simulink model "Boeing787_NewMission_ElectricalThermalHydraulicECS"  (R2016a)
settings: Solver=ode23tb  SolverMode=SingleTasking  StartTime=0.0  StopTime=346  RelTol=1e-3
InitFcn:
  | load('SampleOutput.mat')
  | 
  | load('SampleFuelBurn.mat')
undefined symbols (not defined in the file): ailerons, AirProp, B_737, CurrentMission, elevator, FuelBurn, HydProp, landing_gear, rudder, seed, thrust_rev
libraries: PowerFlowLib x68, simulink x20, powerlib_meascontrol x1
(part 18 of 24)

== system Boeing787_NewMission_ElectricalThermalHydraulicECS/Hydraulic/Center Hydraulic System/Bootstrap Reservoir1 ==
  Piston Pressure : Inport
  Bypass Return : Inport  Port=2
  mdot_out : Inport  Port=3
  Return : Inport  Port=4
  Add : Sum  Inputs=+-
  Bleed Valve on/off : Switch  Criteria=u2 ~= 0  ZeroCross=off
  Bleed Valve on/off1 : Switch  Criteria=u2 > Threshold  ZeroCross=off
  Bus Creator : BusCreator  Inputs=2
  Bus Creator1 : BusCreator  Inputs=3
  Bus Creator2 : BusCreator  Inputs=3
  Bus Selector2 : BusSelector  OutputSignals=pres_kPa
  Bus Selector3 : BusSelector  OutputSignals=temp_K,mdot_kgps
  Bus Selector4 : BusSelector  OutputSignals=pres_kPa,mdot_kgps,temp_K
  Divide : Product  Inputs=****/
  Divide1 : Product  Inputs=**/
  Divide2 : Product  Inputs=/*
  Divide3 : Product  Inputs=**
  Divide4 : Product  Inputs=**
  Gain : Gain  Gain=1/1000
  Gain1 : Gain  Gain=pres_loss/100
  Gain{2..7} (6 alike) : Gain
  R_air : Constant  Value=286.9
  Relational Operator : RelationalOperator  OutDataTypeStr=boolean
  Sum : Sum  Inputs=++-
  Sum of Elements : Sum  Inputs=+
  Sum1 : Sum  Inputs=|+-
  Sum2 : Sum  Inputs=-+|
  Sum3 : Sum  Inputs=-+|
  Sum4 : Sum  Inputs=|++
  Temp : Integrator  InitialCondition=T_init  LimitOutput=on  LowerSaturationLimit=eps
  Terminator : Terminator
  Terminator1 : Terminator
  Z(T,P) : Lookup_n-D  BreakpointsForDimension1=AirProp.T2  BreakpointsForDimension2=AirProp.P2  Table=AirProp.Z  RndMeth=Simplest  InputSameDT=on
  air pres : Integrator  InitialCondition=P_init*1000
  mass : Integrator  InitialCondition=mass_init  LimitOutput=on  LowerSaturationLimit=eps
  mass flow off{,1,7..9} (5 alike) : Constant  Value=0
  mass flow off10 : Constant  Value=T_init
  mass flow off2 : Constant  Value=High_Pres_Area
  mass flow off3 : Constant  Value=Low_Pres_Area
  mass flow off4 : Constant  Value=10
  mass flow off5 : Constant  Value=275.79
  mass flow off6 : Constant  Value=-10
  resevor volume : Constant  Value=res_vol
  rho(T) : Lookup_n-D  NumberOfTableDimensions=1  BreakpointsForDimension1=HydProp.T  Table=HydProp.rho_T  RndMeth=Simplest  InputSameDT=on
  Fluid Conditions : Outport
  wires:
  Piston Pressure/1 -> Sum4/1, Divide3/1
  mass flow off1/1 -> Bleed Valve on/off/3
  Divide2/1 -> Sum1/2
  rho(T)/1 -> Divide2/1
  Sum of Elements/1 -> Sum/2
  Return/1 -> Sum of Elements/1
  mass flow off10/1 -> Gain5/1
  Temp/1 -> rho(T)/1, Sum3/1  "temp_K"
  Sum3/1 -> Divide1/1
  Divide1/1 -> Temp/1
  mass/1 -> Divide1/3, Divide2/2
  Bus Creator1/1 -> Fluid Conditions/1
  [valve_cmd] -> Bleed Valve on/off/2
  Relational Operator/1 -> [valve_cmd]
  mass flow off/1 -> Bleed Valve on/off/1
  Bus Selector2/1 -> Relational Operator/1  "<pres_kPa>"
  Bus Selector4/1 -> Relational Operator/2  "<pres_kPa>"
  Bleed Valve on/off/1 -> Terminator1/1, Gain1/1, Sum2/2
  Bus Selector4/2 -> Terminator/1  "<mdot_kgps>"
  Sum2/1 -> Divide/2  "dm/dt"
  Bus Creator/1 -> Bus Selector2/1
  Gain1/1 -> Sum2/1, Bus Creator/1  "mdot_kgps"
  Gain/1 -> Bus Creator/2, Z(T,P)/2  "pres_kPa"
  Sum1/1 -> Divide/5
  resevor volume/1 -> Sum1/1
  air pres/1 -> Gain/1
  Divide/1 -> air pres/1
  Z(T,P)/1 -> Divide/4
  R_air/1 -> Divide/1
  Bus Selector4/3 -> Divide/3, Z(T,P)/1  "<temp_K>"
  Sum/1 -> mass/1  "dm/dt"
  mdot_out/1 -> Gain6/1, Sum/3  "mdot_kgps"
  Bus Selector3/2 -> Sum/1, Divide1/2  "<mdot_kgps>"
  Bypass Return/1 -> Bus Selector3/1
  mass flow off2/1 -> Divide3/2
  mass flow off3/1 -> Divide4/2
  mass flow off5/1 -> Divide4/1
  Divide4/1 -> Add/2
  Divide3/1 -> Add/1
  Add/1 -> Bleed Valve on/off1/2
  mass flow off6/1 -> Bleed Valve on/off1/3
  Bleed Valve on/off1/1 -> Sum4/2
  mass flow off4/1 -> Bleed Valve on/off1/1  "pres_kPa"
  Bus Creator2/1 -> Bus Selector4/1
  mass flow off9/1 -> Gain4/1
  mass flow off8/1 -> Gain3/1
  mass flow off7/1 -> Gain2/1
  Gain2/1 -> Bus Creator2/1  "pres_kPa"
  Gain4/1 -> Bus Creator2/3  "temp_K"
  Gain3/1 -> Bus Creator2/2  "mdot_kgps"
  Gain6/1 -> Bus Creator1/3  "mdot_kgps"
  Gain5/1 -> Bus Creator1/2  "temp_K"
  Sum4/1 -> Gain7/1  "pres_kPa"
  Gain7/1 -> Bus Creator1/1  "pres_kPa"

== system Boeing787_NewMission_ElectricalThermalHydraulicECS/Hydraulic/Center Hydraulic System/Bootstrap Reservoir2 ==
  Piston Pressure : Inport
  Bypass Return : Inport  Port=2
  mdot_out : Inport  Port=3
  Return : Inport  Port=4
  Add : Sum  Inputs=+-
  Bleed Valve on/off : Switch  Criteria=u2 ~= 0  ZeroCross=off
  Bleed Valve on/off1 : Switch  Criteria=u2 > Threshold  ZeroCross=off
  Bus Creator : BusCreator  Inputs=2
  Bus Creator1 : BusCreator  Inputs=3
  Bus Creator2 : BusCreator  Inputs=3
  Bus Selector2 : BusSelector  OutputSignals=pres_kPa
  Bus Selector3 : BusSelector  OutputSignals=temp_K,mdot_kgps
  Bus Selector4 : BusSelector  OutputSignals=pres_kPa,mdot_kgps,temp_K
  Divide : Product  Inputs=****/
  Divide1 : Product  Inputs=**/
  Divide2 : Product  Inputs=/*
  Divide3 : Product  Inputs=**
  Divide4 : Product  Inputs=**
  Gain : Gain  Gain=1/1000
  Gain1 : Gain  Gain=pres_loss/100
  Gain{2..7} (6 alike) : Gain
  R_air : Constant  Value=286.9
  Relational Operator : RelationalOperator  OutDataTypeStr=boolean
  Sum : Sum  Inputs=++-
  Sum of Elements : Sum  Inputs=+
  Sum1 : Sum  Inputs=|+-
  Sum2 : Sum  Inputs=-+|
  Sum3 : Sum  Inputs=-+|
  Sum4 : Sum  Inputs=|++
  Temp : Integrator  InitialCondition=T_init  LimitOutput=on  LowerSaturationLimit=eps
  Terminator : Terminator
  Terminator1 : Terminator
  Z(T,P) : Lookup_n-D  BreakpointsForDimension1=AirProp.T2  BreakpointsForDimension2=AirProp.P2  Table=AirProp.Z  RndMeth=Simplest  InputSameDT=on
  air pres : Integrator  InitialCondition=P_init*1000
  mass : Integrator  InitialCondition=mass_init  LimitOutput=on  LowerSaturationLimit=eps
  mass flow off{,1,7..9} (5 alike) : Constant  Value=0
  mass flow off2 : Constant  Value=High_Pres_Area
  mass flow off3 : Constant  Value=Low_Pres_Area
  mass flow off4 : Constant  Value=10
  mass flow off5 : Constant  Value=275.79
  mass flow off6 : Constant  Value=-10
  resevor volume : Constant  Value=res_vol
  rho(T) : Lookup_n-D  NumberOfTableDimensions=1  BreakpointsForDimension1=HydProp.T  Table=HydProp.rho_T  RndMeth=Simplest  InputSameDT=on
  Fluid Conditions : Outport
  wires:
  Piston Pressure/1 -> Sum4/1, Divide3/1
  mass flow off1/1 -> Bleed Valve on/off/3
  Divide2/1 -> Sum1/2
  rho(T)/1 -> Divide2/1
  Sum of Elements/1 -> Sum/2
  Return/1 -> Sum of Elements/1
  Bus Selector3/1 -> Gain5/1  "<temp_K>"
  Temp/1 -> rho(T)/1, Sum3/1  "temp_K"
  Sum3/1 -> Divide1/1
  Divide1/1 -> Temp/1
  mass/1 -> Divide1/3, Divide2/2
  Bus Creator1/1 -> Fluid Conditions/1
  [valve_cmd] -> Bleed Valve on/off/2
  Relational Operator/1 -> [valve_cmd]
  mass flow off/1 -> Bleed Valve on/off/1
  Bus Selector2/1 -> Relational Operator/1  "<pres_kPa>"
  Bus Selector4/1 -> Relational Operator/2  "<pres_kPa>"
  Bleed Valve on/off/1 -> Terminator1/1, Gain1/1, Sum2/2
  Bus Selector4/2 -> Terminator/1  "<mdot_kgps>"
  Sum2/1 -> Divide/2  "dm/dt"
  Bus Creator/1 -> Bus Selector2/1
  Gain1/1 -> Sum2/1, Bus Creator/1  "mdot_kgps"
  Gain/1 -> Bus Creator/2, Z(T,P)/2  "pres_kPa"
  Sum1/1 -> Divide/5
  resevor volume/1 -> Sum1/1
  air pres/1 -> Gain/1
  Divide/1 -> air pres/1
  Z(T,P)/1 -> Divide/4
  R_air/1 -> Divide/1
  Bus Selector4/3 -> Divide/3, Z(T,P)/1  "<temp_K>"
  Sum/1 -> mass/1  "dm/dt"
  mdot_out/1 -> Gain6/1, Sum/3  "mdot_kgps"
  Bus Selector3/2 -> Sum/1, Divide1/2  "<mdot_kgps>"
  Bypass Return/1 -> Bus Selector3/1
  mass flow off2/1 -> Divide3/2
  mass flow off3/1 -> Divide4/2
  mass flow off5/1 -> Divide4/1
  Divide4/1 -> Add/2
  Divide3/1 -> Add/1
  Add/1 -> Bleed Valve on/off1/2
  mass flow off6/1 -> Bleed Valve on/off1/3
  Bleed Valve on/off1/1 -> Sum4/2
  mass flow off4/1 -> Bleed Valve on/off1/1  "pres_kPa"
  Bus Creator2/1 -> Bus Selector4/1
  mass flow off9/1 -> Gain4/1
  mass flow off8/1 -> Gain3/1
  mass flow off7/1 -> Gain2/1
  Gain2/1 -> Bus Creator2/1  "pres_kPa"
  Gain4/1 -> Bus Creator2/3  "temp_K"
  Gain3/1 -> Bus Creator2/2  "mdot_kgps"
  Gain6/1 -> Bus Creator1/3  "mdot_kgps"
  Gain5/1 -> Bus Creator1/2  "temp_K"
  Sum4/1 -> Gain7/1  "pres_kPa"
  Gain7/1 -> Bus Creator1/1  "pres_kPa"

== system Boeing787_NewMission_ElectricalThermalHydraulicECS/Hydraulic/Center Hydraulic System/DC Speed Servo ==
  T_load (Nm) : Inport
  Speed_ref (RPM) : Inport  Port=2
  Voltage : Inport  Port=3
  DC Machine : Subsystem
  Fcn : Fcn  Expr=u(1)/(u(2)+0.1)
  Gain2 : Gain  Gain=60/(2*pi)
  Mux : Mux  Inputs=2
  PID Controller : simulink/Continuous/PID Controller  Controller=PID  TimeDomain=Continuous-time  SampleTime=-1  IntegratorMethod=Forward Euler  FilterMethod=Forward Euler  Form=Parallel  UseFilter=on  ControllerParametersSource=internal  P=1  I=0.1  D=0  N=100  InitialConditionSource=internal  InitialConditionForIntegrator=0  InitialConditionForFilter=0  ExternalReset=none  LimitOutput=off  UpperSaturationLimit=inf  LowerSaturationLimit=-inf  LinearizeAsGain=on  AntiWindupMode=none  Kb=1  TrackingMode=off  Kt=1  PParamMin=[]  PParamMax=[]  IParamMin=[]  IParamMax=[]  DParamMin=[]  DParamMax=[]  NParamMin=[]  NParamMax=[]  KbParamMin=[]  KbParamMax=[]  KtParamMin=[]  KtParamMax=[]  POutMin=[]  POutMax=[]  IOutMin=[]  IOutMax=[]  DOutMin=[]  DOutMax=[]  NOutMin=[]  NOutMax=[]  KbOutMin=[]  KbOutMax=[]  KtOutMin=[]  KtOutMax=[]  IntegratorOutMin=[]  IntegratorOutMax=[]  FilterOutMin=[]  FilterOutMax=[]  SumOutMin=[]  SumOutMax=[]  SumI1OutMin=[]  SumI1OutMax=[]  SumI2OutMin=[]  SumI2OutMax=[]  SumI3OutMin=[]  SumI3OutMax=[]  SumDOutMin=[]  SumDOutMax=[]  SaturationOutMin=[]  SaturationOutMax=[]  IntegratorContinuousStateAttributes=''  IntegratorStateMustResolveToSignalObject=off  IntegratorRTWStateStorageClass=Auto  FilterContinuousStateAttributes=''  FilterStateMustResolveToSignalObject=off  FilterRTWStateStorageClass=Auto  DifferentiatorICPrevScaledInput=0  DifferentiatorOutMin=[]  DifferentiatorOutMax=[]
  Sum : Sum  Inputs=-+|
  Terminator{,1..3} (4 alike) : Terminator
  w_m : Outport
  i_load : Outport  Port=2
  T_em : Outport  Port=3
  Ploss : Outport  Port=4
  wires:
  DC Machine/5(Plosses) -> Ploss/1
  Sum/1 -> PID Controller/1
  Gain2/1 -> Sum/1, w_m/1
  Speed_ref (RPM)/1 -> Sum/2
  T_load (Nm)/1 -> DC Machine/3(Tload)
  DC Machine/6(Te) -> T_em/1
  Mux/1 -> Fcn/1
  DC Machine/3(Pe) -> Mux/1
  Fcn/1 -> i_load/1
  DC Machine/7(Speed) -> Gain2/1
  Voltage/1 -> DC Machine/1(Vf), Mux/2
  PID Controller/1 -> DC Machine/2(Va)
  DC Machine/1(If) -> Terminator/1
  DC Machine/2(Ia) -> Terminator1/1
  DC Machine/4(Pm) -> Terminator2/1
  DC Machine/8(theta) -> Terminator3/1

== system Boeing787_NewMission_ElectricalThermalHydraulicECS/Hydraulic/Center Hydraulic System/DC Speed Servo1 ==
  T_load (Nm) : Inport
  Speed_ref (RPM) : Inport  Port=2
  Voltage : Inport  Port=3
  DC Machine : Subsystem
  Fcn : Fcn  Expr=u(1)/(u(2)+0.1)
  Gain2 : Gain  Gain=60/(2*pi)
  Mux : Mux  Inputs=2
  PID Controller : simulink/Continuous/PID Controller  Controller=PID  TimeDomain=Continuous-time  SampleTime=-1  IntegratorMethod=Forward Euler  FilterMethod=Forward Euler  Form=Parallel  UseFilter=on  ControllerParametersSource=internal  P=1  I=0.1  D=0  N=100  InitialConditionSource=internal  InitialConditionForIntegrator=0  InitialConditionForFilter=0  ExternalReset=none  LimitOutput=off  UpperSaturationLimit=inf  LowerSaturationLimit=-inf  LinearizeAsGain=on  AntiWindupMode=none  Kb=1  TrackingMode=off  Kt=1  PParamMin=[]  PParamMax=[]  IParamMin=[]  IParamMax=[]  DParamMin=[]  DParamMax=[]  NParamMin=[]  NParamMax=[]  KbParamMin=[]  KbParamMax=[]  KtParamMin=[]  KtParamMax=[]  POutMin=[]  POutMax=[]  IOutMin=[]  IOutMax=[]  DOutMin=[]  DOutMax=[]  NOutMin=[]  NOutMax=[]  KbOutMin=[]  KbOutMax=[]  KtOutMin=[]  KtOutMax=[]  IntegratorOutMin=[]  IntegratorOutMax=[]  FilterOutMin=[]  FilterOutMax=[]  SumOutMin=[]  SumOutMax=[]  SumI1OutMin=[]  SumI1OutMax=[]  SumI2OutMin=[]  SumI2OutMax=[]  SumI3OutMin=[]  SumI3OutMax=[]  SumDOutMin=[]  SumDOutMax=[]  SaturationOutMin=[]  SaturationOutMax=[]  IntegratorContinuousStateAttributes=''  IntegratorStateMustResolveToSignalObject=off  IntegratorRTWStateStorageClass=Auto  FilterContinuousStateAttributes=''  FilterStateMustResolveToSignalObject=off  FilterRTWStateStorageClass=Auto  DifferentiatorICPrevScaledInput=0  DifferentiatorOutMin=[]  DifferentiatorOutMax=[]
  Sum : Sum  Inputs=-+|
  Terminator{,1..3} (4 alike) : Terminator
  w_m : Outport
  i_load : Outport  Port=2
  T_em : Outport  Port=3
  Ploss : Outport  Port=4
  wires:
  DC Machine/5(Plosses) -> Ploss/1
  Sum/1 -> PID Controller/1
  Gain2/1 -> Sum/1, w_m/1
  Speed_ref (RPM)/1 -> Sum/2
  T_load (Nm)/1 -> DC Machine/3(Tload)
  DC Machine/6(Te) -> T_em/1
  Mux/1 -> Fcn/1
  DC Machine/3(Pe) -> Mux/1
  Fcn/1 -> i_load/1
  DC Machine/7(Speed) -> Gain2/1
  Voltage/1 -> DC Machine/1(Vf), Mux/2
  PID Controller/1 -> DC Machine/2(Va)
  DC Machine/1(If) -> Terminator3/1
  DC Machine/2(Ia) -> Terminator2/1
  DC Machine/4(Pm) -> Terminator1/1
  DC Machine/8(theta) -> Terminator/1

== system Boeing787_NewMission_ElectricalThermalHydraulicECS/Hydraulic/Center Hydraulic System/Sinks ==
  "Motor PLoss 1 " : Inport
  Motor PLoss 2 : Inport  Port=2
  Motor Current Load 1 : Inport  Port=3
  Motor Current Load 2 : Inport  Port=4
  Out1 : Outport
  wires:
  "Motor PLoss 1 "/1 -> Out1/1

== system Boeing787_NewMission_ElectricalThermalHydraulicECS/Hydraulic/Left Hydraulic System/Bootstrap Reservoir ==
  Piston Pressure : Inport
  Bypass Return : Inport  Port=2
  mdot_out : Inport  Port=3
  Return : Inport  Port=4
  Add : Sum  Inputs=+-
  Bleed Valve on/off : Switch  Criteria=u2 ~= 0  ZeroCross=off
  Bleed Valve on/off1 : Switch  Criteria=u2 > Threshold  ZeroCross=off
  Bus Creator : BusCreator  Inputs=2
  Bus Creator1 : BusCreator  Inputs=3
  Bus Creator2 : BusCreator  Inputs=3
  Bus Selector2 : BusSelector  OutputSignals=pres_kPa
  Bus Selector3 : BusSelector  OutputSignals=temp_K,mdot_kgps
  Bus Selector4 : BusSelector  OutputSignals=pres_kPa,mdot_kgps,temp_K
  Divide : Product  Inputs=****/
  Divide1 : Product  Inputs=**/
  Divide2 : Product  Inputs=/*
  Divide3 : Product  Inputs=**
  Divide4 : Product  Inputs=**
  Gain : Gain  Gain=1/1000
  Gain1 : Gain  Gain=pres_loss/100
  Gain{2..7} (6 alike) : Gain
  R_air : Constant  Value=286.9
  Relational Operator : RelationalOperator  OutDataTypeStr=boolean
  Sum : Sum  Inputs=++-
  Sum of Elements : Sum  Inputs=+
  Sum1 : Sum  Inputs=|+-
  Sum2 : Sum  Inputs=-+|
  Sum3 : Sum  Inputs=-+|
  Sum4 : Sum  Inputs=|++
  Temp : Integrator  InitialCondition=T_init  LimitOutput=on  LowerSaturationLimit=eps
  Terminator : Terminator
  Terminator1 : Terminator
  Z(T,P) : Lookup_n-D  BreakpointsForDimension1=AirProp.T2  BreakpointsForDimension2=AirProp.P2  Table=AirProp.Z  RndMeth=Simplest  InputSameDT=on
  air pres : Integrator  InitialCondition=P_init*1000
  mass : Integrator  InitialCondition=mass_init  LimitOutput=on  LowerSaturationLimit=eps
  mass flow off{,1,7..9} (5 alike) : Constant  Value=0
  mass flow off2 : Constant  Value=High_Pres_Area
  mass flow off3 : Constant  Value=Low_Pres_Area
  mass flow off4 : Constant  Value=10
  mass flow off5 : Constant  Value=275.79
  mass flow off6 : Constant  Value=-10
  resevor volume : Constant  Value=res_vol
  rho(T) : Lookup_n-D  NumberOfTableDimensions=1  BreakpointsForDimension1=HydProp.T  Table=HydProp.rho_T  RndMeth=Simplest  InputSameDT=on
  Fluid Conditions : Outport
  wires:
  Piston Pressure/1 -> Sum4/1, Divide3/1
  mass flow off1/1 -> Bleed Valve on/off/3
  Divide2/1 -> Sum1/2
  rho(T)/1 -> Divide2/1
  Sum of Elements/1 -> Sum/2
  Return/1 -> Sum of Elements/1
  Bus Selector3/1 -> Gain5/1  "<temp_K>"
  Temp/1 -> rho(T)/1, Sum3/1  "temp_K"
  Sum3/1 -> Divide1/1
  Divide1/1 -> Temp/1
  mass/1 -> Divide1/3, Divide2/2
  Bus Creator1/1 -> Fluid Conditions/1
  [valve_cmd] -> Bleed Valve on/off/2
  Relational Operator/1 -> [valve_cmd]
  mass flow off/1 -> Bleed Valve on/off/1
  Bus Selector2/1 -> Relational Operator/1  "<pres_kPa>"
  Bus Selector4/1 -> Relational Operator/2  "<pres_kPa>"
  Bleed Valve on/off/1 -> Terminator1/1, Gain1/1, Sum2/2
  Bus Selector4/2 -> Terminator/1  "<mdot_kgps>"
  Sum2/1 -> Divide/2  "dm/dt"
  Bus Creator/1 -> Bus Selector2/1
  Gain1/1 -> Sum2/1, Bus Creator/1  "mdot_kgps"
  Gain/1 -> Bus Creator/2, Z(T,P)/2  "pres_kPa"
  Sum1/1 -> Divide/5
  resevor volume/1 -> Sum1/1
  air pres/1 -> Gain/1
  Divide/1 -> air pres/1
  Z(T,P)/1 -> Divide/4
  R_air/1 -> Divide/1
  Bus Selector4/3 -> Divide/3, Z(T,P)/1  "<temp_K>"
  Sum/1 -> mass/1  "dm/dt"
  mdot_out/1 -> Gain6/1, Sum/3  "mdot_kgps"
  Bus Selector3/2 -> Sum/1, Divide1/2  "<mdot_kgps>"
  Bypass Return/1 -> Bus Selector3/1
  mass flow off2/1 -> Divide3/2
  mass flow off3/1 -> Divide4/2
  mass flow off5/1 -> Divide4/1
  Divide4/1 -> Add/2
  Divide3/1 -> Add/1
  Add/1 -> Bleed Valve on/off1/2
  mass flow off6/1 -> Bleed Valve on/off1/3
  Bleed Valve on/off1/1 -> Sum4/2
  mass flow off4/1 -> Bleed Valve on/off1/1  "pres_kPa"
  Bus Creator2/1 -> Bus Selector4/1
  mass flow off9/1 -> Gain4/1
  mass flow off8/1 -> Gain3/1
  mass flow off7/1 -> Gain2/1
  Gain2/1 -> Bus Creator2/1  "pres_kPa"
  Gain4/1 -> Bus Creator2/3  "temp_K"
  Gain3/1 -> Bus Creator2/2  "mdot_kgps"
  Gain7/1 -> Bus Creator1/1  "pres_kPa"
  Gain6/1 -> Bus Creator1/3  "mdot_kgps"
  Gain5/1 -> Bus Creator1/2  "temp_K"
  Sum4/1 -> Gain7/1  "pres_kPa"

== system Boeing787_NewMission_ElectricalThermalHydraulicECS/Hydraulic/Left Hydraulic System/Bootstrap Reservoir1 ==
  Piston Pressure : Inport
  Bypass Return : Inport  Port=2
  mdot_out : Inport  Port=3
  Return : Inport  Port=4
  Add : Sum  Inputs=+-
  Bleed Valve on/off : Switch  Criteria=u2 ~= 0  ZeroCross=off
  Bleed Valve on/off1 : Switch  Criteria=u2 > Threshold  ZeroCross=off
  Bus Creator : BusCreator  Inputs=2
  Bus Creator1 : BusCreator  Inputs=3
  Bus Creator2 : BusCreator  Inputs=3
  Bus Selector2 : BusSelector  OutputSignals=pres_kPa
  Bus Selector3 : BusSelector  OutputSignals=temp_K,mdot_kgps
  Bus Selector4 : BusSelector  OutputSignals=pres_kPa,mdot_kgps,temp_K
  Divide : Product  Inputs=****/
  Divide1 : Product  Inputs=**/
  Divide2 : Product  Inputs=/*
  Divide3 : Product  Inputs=**
  Divide4 : Product  Inputs=**
  Gain : Gain  Gain=1/1000
  Gain1 : Gain  Gain=pres_loss/100
  Gain{2..7} (6 alike) : Gain
  R_air : Constant  Value=286.9
  Relational Operator : RelationalOperator  OutDataTypeStr=boolean
  Sum : Sum  Inputs=++-
  Sum of Elements : Sum  Inputs=+
  Sum1 : Sum  Inputs=|+-
  Sum2 : Sum  Inputs=-+|
  Sum3 : Sum  Inputs=-+|
  Sum4 : Sum  Inputs=|++
  Temp : Integrator  InitialCondition=T_init  LimitOutput=on  LowerSaturationLimit=eps
  Terminator : Terminator
  Terminator1 : Terminator
  Z(T,P) : Lookup_n-D  BreakpointsForDimension1=AirProp.T2  BreakpointsForDimension2=AirProp.P2  Table=AirProp.Z  RndMeth=Simplest  InputSameDT=on
  air pres : Integrator  InitialCondition=P_init*1000
  mass : Integrator  InitialCondition=mass_init  LimitOutput=on  LowerSaturationLimit=eps
  mass flow off{,1,7..9} (5 alike) : Constant  Value=0
  mass flow off10 : Constant  Value=T_init
  mass flow off2 : Constant  Value=High_Pres_Area
  mass flow off3 : Constant  Value=Low_Pres_Area
  mass flow off4 : Constant  Value=10
  mass flow off5 : Constant  Value=275.79
  mass flow off6 : Constant  Value=-10
  resevor volume : Constant  Value=res_vol
  rho(T) : Lookup_n-D  NumberOfTableDimensions=1  BreakpointsForDimension1=HydProp.T  Table=HydProp.rho_T  RndMeth=Simplest  InputSameDT=on
  Fluid Conditions : Outport
  wires:
  Piston Pressure/1 -> Sum4/1, Divide3/1
  mass flow off1/1 -> Bleed Valve on/off/3
  Divide2/1 -> Sum1/2
  rho(T)/1 -> Divide2/1
  Sum of Elements/1 -> Sum/2
  Return/1 -> Sum of Elements/1
  mass flow off10/1 -> Gain5/1
  Temp/1 -> rho(T)/1, Sum3/1  "temp_K"
  Sum3/1 -> Divide1/1
  Divide1/1 -> Temp/1
  mass/1 -> Divide1/3, Divide2/2
  Bus Creator1/1 -> Fluid Conditions/1
  [valve_cmd] -> Bleed Valve on/off/2
  Relational Operator/1 -> [valve_cmd]
  mass flow off/1 -> Bleed Valve on/off/1
  Bus Selector2/1 -> Relational Operator/1  "<pres_kPa>"
  Bus Selector4/1 -> Relational Operator/2  "<pres_kPa>"
  Bleed Valve on/off/1 -> Terminator1/1, Gain1/1, Sum2/2
  Bus Selector4/2 -> Terminator/1  "<mdot_kgps>"
  Sum2/1 -> Divide/2  "dm/dt"
  Bus Creator/1 -> Bus Selector2/1
  Gain1/1 -> Sum2/1, Bus Creator/1  "mdot_kgps"
  Gain/1 -> Bus Creator/2, Z(T,P)/2  "pres_kPa"
  Sum1/1 -> Divide/5
  resevor volume/1 -> Sum1/1
  air pres/1 -> Gain/1
  Divide/1 -> air pres/1
  Z(T,P)/1 -> Divide/4
  R_air/1 -> Divide/1
  Bus Selector4/3 -> Divide/3, Z(T,P)/1  "<temp_K>"
  Sum/1 -> mass/1  "dm/dt"
  mdot_out/1 -> Gain6/1, Sum/3  "mdot_kgps"
  Bus Selector3/2 -> Sum/1, Divide1/2  "<mdot_kgps>"
  Bypass Return/1 -> Bus Selector3/1
  mass flow off2/1 -> Divide3/2
  mass flow off3/1 -> Divide4/2
  mass flow off5/1 -> Divide4/1
  Divide4/1 -> Add/2
  Divide3/1 -> Add/1
  Add/1 -> Bleed Valve on/off1/2
  mass flow off6/1 -> Bleed Valve on/off1/3
  Bleed Valve on/off1/1 -> Sum4/2
  mass flow off4/1 -> Bleed Valve on/off1/1  "pres_kPa"
  Bus Creator2/1 -> Bus Selector4/1
  mass flow off9/1 -> Gain4/1
  mass flow off8/1 -> Gain3/1
  mass flow off7/1 -> Gain2/1
  Gain2/1 -> Bus Creator2/1  "pres_kPa"
  Gain4/1 -> Bus Creator2/3  "temp_K"
  Gain3/1 -> Bus Creator2/2  "mdot_kgps"
  Gain7/1 -> Bus Creator1/1  "pres_kPa"
  Gain6/1 -> Bus Creator1/3  "mdot_kgps"
  Gain5/1 -> Bus Creator1/2  "temp_K"
  Sum4/1 -> Gain7/1  "pres_kPa"

== system Boeing787_NewMission_ElectricalThermalHydraulicECS/Hydraulic/Left Hydraulic System/DC Speed Servo ==
  T_load (Nm) : Inport
  Speed_ref (RPM) : Inport  Port=2
  Voltage : Inport  Port=3
  DC Machine : Subsystem
  Fcn : Fcn  Expr=u(1)/(u(2)+0.1)
  Gain2 : Gain  Gain=60/(2*pi)
  Mux : Mux  Inputs=2
  PID Controller : simulink/Continuous/PID Controller  Controller=PID  TimeDomain=Continuous-time  SampleTime=-1  IntegratorMethod=Forward Euler  FilterMethod=Forward Euler  Form=Parallel  UseFilter=on  ControllerParametersSource=internal  P=1  I=0.1  D=0  N=100  InitialConditionSource=internal  InitialConditionForIntegrator=0  InitialConditionForFilter=0  ExternalReset=none  LimitOutput=off  UpperSaturationLimit=inf  LowerSaturationLimit=-inf  LinearizeAsGain=on  AntiWindupMode=none  Kb=1  TrackingMode=off  Kt=1  PParamMin=[]  PParamMax=[]  IParamMin=[]  IParamMax=[]  DParamMin=[]  DParamMax=[]  NParamMin=[]  NParamMax=[]  KbParamMin=[]  KbParamMax=[]  KtParamMin=[]  KtParamMax=[]  POutMin=[]  POutMax=[]  IOutMin=[]  IOutMax=[]  DOutMin=[]  DOutMax=[]  NOutMin=[]  NOutMax=[]  KbOutMin=[]  KbOutMax=[]  KtOutMin=[]  KtOutMax=[]  IntegratorOutMin=[]  IntegratorOutMax=[]  FilterOutMin=[]  FilterOutMax=[]  SumOutMin=[]  SumOutMax=[]  SumI1OutMin=[]  SumI1OutMax=[]  SumI2OutMin=[]  SumI2OutMax=[]  SumI3OutMin=[]  SumI3OutMax=[]  SumDOutMin=[]  SumDOutMax=[]  SaturationOutMin=[]  SaturationOutMax=[]  IntegratorContinuousStateAttributes=''  IntegratorStateMustResolveToSignalObject=off  IntegratorRTWStateStorageClass=Auto  FilterContinuousStateAttributes=''  FilterStateMustResolveToSignalObject=off  FilterRTWStateStorageClass=Auto  DifferentiatorICPrevScaledInput=0  DifferentiatorOutMin=[]  DifferentiatorOutMax=[]
  Sum : Sum  Inputs=-+|
  Terminator{,1..3} (4 alike) : Terminator
  w_m : Outport
  i_load : Outport  Port=2
  T_em : Outport  Port=3
  Ploss : Outport  Port=4
  wires:
  DC Machine/5(Plosses) -> Ploss/1
  Sum/1 -> PID Controller/1
  Gain2/1 -> Sum/1, w_m/1
  Speed_ref (RPM)/1 -> Sum/2
  T_load (Nm)/1 -> DC Machine/3(Tload)
  DC Machine/6(Te) -> T_em/1
  Mux/1 -> Fcn/1
  DC Machine/3(Pe) -> Mux/1
  Fcn/1 -> i_load/1
  DC Machine/7(Speed) -> Gain2/1
  Voltage/1 -> DC Machine/1(Vf), Mux/2
  PID Controller/1 -> DC Machine/2(Va)
  DC Machine/1(If) -> Terminator/1
  DC Machine/2(Ia) -> Terminator1/1
  DC Machine/4(Pm) -> Terminator2/1
  DC Machine/8(theta) -> Terminator3/1

== system Boeing787_NewMission_ElectricalThermalHydraulicECS/Hydraulic/Left Hydraulic System/Sinks ==
  "Motor PLoss " : Inport
  Motor Current Load : Inport  Port=2
  Out1 : Outport
  wires:
  "Motor PLoss "/1 -> Out1/1

== system Boeing787_NewMission_ElectricalThermalHydraulicECS/Hydraulic/Right Hydraulic System/Bootstrap Reservoir ==
  Piston Pressure : Inport
  Bypass Return : Inport  Port=2
  mdot_out : Inport  Port=3
  Return : Inport  Port=4
  Add : Sum  Inputs=+-
  Bleed Valve on/off : Switch  Criteria=u2 ~= 0  ZeroCross=off
  Bleed Valve on/off1 : Switch  Criteria=u2 > Threshold  ZeroCross=off
  Bus Creator : BusCreator  Inputs=2
  Bus Creator1 : BusCreator  Inputs=3
  Bus Creator2 : BusCreator  Inputs=3
  Bus Selector2 : BusSelector  OutputSignals=pres_kPa
  Bus Selector3 : BusSelector  OutputSignals=temp_K,mdot_kgps
  Bus Selector4 : BusSelector  OutputSignals=pres_kPa,mdot_kgps,temp_K
  Divide : Product  Inputs=****/
  Divide1 : Product  Inputs=**/
  Divide2 : Product  Inputs=/*
  Divide3 : Product  Inputs=**
  Divide4 : Product  Inputs=**
  Gain : Gain  Gain=1/1000
  Gain1 : Gain  Gain=pres_loss/100
  Gain{2..7} (6 alike) : Gain
  R_air : Constant  Value=286.9
  Relational Operator : RelationalOperator  OutDataTypeStr=boolean
  Sum : Sum  Inputs=++-
  Sum of Elements : Sum  Inputs=+
  Sum1 : Sum  Inputs=|+-
  Sum2 : Sum  Inputs=-+|
  Sum3 : Sum  Inputs=-+|
  Sum4 : Sum  Inputs=|++
  Temp : Integrator  InitialCondition=T_init  LimitOutput=on  LowerSaturationLimit=eps
  Terminator : Terminator
  Terminator1 : Terminator
  Z(T,P) : Lookup_n-D  BreakpointsForDimension1=AirProp.T2  BreakpointsForDimension2=AirProp.P2  Table=AirProp.Z  RndMeth=Simplest  InputSameDT=on
  air pres : Integrator  InitialCondition=P_init*1000
  mass : Integrator  InitialCondition=mass_init  LimitOutput=on  LowerSaturationLimit=eps
  mass flow off{,1,7..9} (5 alike) : Constant  Value=0
  mass flow off2 : Constant  Value=High_Pres_Area
  mass flow off3 : Constant  Value=Low_Pres_Area
  mass flow off4 : Constant  Value=10
  mass flow off5 : Constant  Value=275.79
  mass flow off6 : Constant  Value=-10
  resevor volume : Constant  Value=res_vol
  rho(T) : Lookup_n-D  NumberOfTableDimensions=1  BreakpointsForDimension1=HydProp.T  Table=HydProp.rho_T  RndMeth=Simplest  InputSameDT=on
  Fluid Conditions : Outport
  wires:
  Piston Pressure/1 -> Sum4/1, Divide3/1
  mass flow off1/1 -> Bleed Valve on/off/3
  Divide2/1 -> Sum1/2
  rho(T)/1 -> Divide2/1
  Sum of Elements/1 -> Sum/2
  Return/1 -> Sum of Elements/1
  Bus Selector3/1 -> Gain5/1  "<temp_K>"
  Temp/1 -> rho(T)/1, Sum3/1  "temp_K"
  Sum3/1 -> Divide1/1
  Divide1/1 -> Temp/1
  mass/1 -> Divide1/3, Divide2/2
  Bus Creator1/1 -> Fluid Conditions/1
  [valve_cmd] -> Bleed Valve on/off/2
  Relational Operator/1 -> [valve_cmd]
  mass flow off/1 -> Bleed Valve on/off/1
  Bus Selector2/1 -> Relational Operator/1  "<pres_kPa>"
  Bus Selector4/1 -> Relational Operator/2  "<pres_kPa>"
  Bleed Valve on/off/1 -> Terminator1/1, Gain1/1, Sum2/2
  Bus Selector4/2 -> Terminator/1  "<mdot_kgps>"
  Sum2/1 -> Divide/2  "dm/dt"
  Bus Creator/1 -> Bus Selector2/1
  Gain1/1 -> Sum2/1, Bus Creator/1  "mdot_kgps"
  Gain/1 -> Bus Creator/2, Z(T,P)/2  "pres_kPa"
  Sum1/1 -> Divide/5
  resevor volume/1 -> Sum1/1
  air pres/1 -> Gain/1
  Divide/1 -> air pres/1
  Z(T,P)/1 -> Divide/4
  R_air/1 -> Divide/1
  Bus Selector4/3 -> Divide/3, Z(T,P)/1  "<temp_K>"
  Sum/1 -> mass/1  "dm/dt"
  mdot_out/1 -> Gain6/1, Sum/3  "mdot_kgps"
  Bus Selector3/2 -> Sum/1, Divide1/2  "<mdot_kgps>"
  Bypass Return/1 -> Bus Selector3/1
  mass flow off2/1 -> Divide3/2
  mass flow off3/1 -> Divide4/2
  mass flow off5/1 -> Divide4/1
  Divide4/1 -> Add/2
  Divide3/1 -> Add/1
  Add/1 -> Bleed Valve on/off1/2
  mass flow off6/1 -> Bleed Valve on/off1/3
  Bleed Valve on/off1/1 -> Sum4/2
  mass flow off4/1 -> Bleed Valve on/off1/1  "pres_kPa"
  Bus Creator2/1 -> Bus Selector4/1
  mass flow off9/1 -> Gain4/1
  mass flow off8/1 -> Gain3/1
  mass flow off7/1 -> Gain2/1
  Gain2/1 -> Bus Creator2/1  "pres_kPa"
  Gain4/1 -> Bus Creator2/3  "temp_K"
  Gain3/1 -> Bus Creator2/2  "mdot_kgps"
  Gain7/1 -> Bus Creator1/1  "pres_kPa"
  Gain6/1 -> Bus Creator1/3  "mdot_kgps"
  Gain5/1 -> Bus Creator1/2  "temp_K"
  Sum4/1 -> Gain7/1  "pres_kPa"

== system Boeing787_NewMission_ElectricalThermalHydraulicECS/Hydraulic/Right Hydraulic System/Bootstrap Reservoir1 ==
  Piston Pressure : Inport
  Bypass Return : Inport  Port=2
  mdot_out : Inport  Port=3
  Return : Inport  Port=4
  Add : Sum  Inputs=+-
  Bleed Valve on/off : Switch  Criteria=u2 ~= 0  ZeroCross=off
  Bleed Valve on/off1 : Switch  Criteria=u2 > Threshold  ZeroCross=off
  Bus Creator : BusCreator  Inputs=2
  Bus Creator1 : BusCreator  Inputs=3
  Bus Creator2 : BusCreator  Inputs=3
  Bus Selector2 : BusSelector  OutputSignals=pres_kPa
  Bus Selector3 : BusSelector  OutputSignals=temp_K,mdot_kgps
  Bus Selector4 : BusSelector  OutputSignals=pres_kPa,mdot_kgps,temp_K
  Divide : Product  Inputs=****/
  Divide1 : Product  Inputs=**/
  Divide2 : Product  Inputs=/*
  Divide3 : Product  Inputs=**
  Divide4 : Product  Inputs=**
  Gain : Gain  Gain=1/1000
  Gain1 : Gain  Gain=pres_loss/100
  Gain{2..7} (6 alike) : Gain
  R_air : Constant  Value=286.9
  Relational Operator : RelationalOperator  OutDataTypeStr=boolean
  Sum : Sum  Inputs=++-
  Sum of Elements : Sum  Inputs=+
  Sum1 : Sum  Inputs=|+-
  Sum2 : Sum  Inputs=-+|
  Sum3 : Sum  Inputs=-+|
  Sum4 : Sum  Inputs=|++
  Temp : Integrator  InitialCondition=T_init  LimitOutput=on  LowerSaturationLimit=eps
  Terminator : Terminator
  Terminator1 : Terminator
  Z(T,P) : Lookup_n-D  BreakpointsForDimension1=AirProp.T2  BreakpointsForDimension2=AirProp.P2  Table=AirProp.Z  RndMeth=Simplest  InputSameDT=on
  air pres : Integrator  InitialCondition=P_init*1000
  mass : Integrator  InitialCondition=mass_init  LimitOutput=on  LowerSaturationLimit=eps
  mass flow off{,1,7..9} (5 alike) : Constant  Value=0
  mass flow off10 : Constant  Value=T_init
  mass flow off2 : Constant  Value=High_Pres_Area
  mass flow off3 : Constant  Value=Low_Pres_Area
  mass flow off4 : Constant  Value=10
  mass flow off5 : Constant  Value=275.79
  mass flow off6 : Constant  Value=-10
  resevor volume : Constant  Value=res_vol
  rho(T) : Lookup_n-D  NumberOfTableDimensions=1  BreakpointsForDimension1=HydProp.T  Table=HydProp.rho_T  RndMeth=Simplest  InputSameDT=on
  Fluid Conditions : Outport
  wires:
  Piston Pressure/1 -> Sum4/1, Divide3/1
  mass flow off1/1 -> Bleed Valve on/off/3
  Divide2/1 -> Sum1/2
  rho(T)/1 -> Divide2/1
  Sum of Elements/1 -> Sum/2
  Return/1 -> Sum of Elements/1
  mass flow off10/1 -> Gain5/1
  Temp/1 -> rho(T)/1, Sum3/1  "temp_K"
  Sum3/1 -> Divide1/1
  Divide1/1 -> Temp/1
  mass/1 -> Divide1/3, Divide2/2
  Bus Creator1/1 -> Fluid Conditions/1
  [valve_cmd] -> Bleed Valve on/off/2
  Relational Operator/1 -> [valve_cmd]
  mass flow off/1 -> Bleed Valve on/off/1
  Bus Selector2/1 -> Relational Operator/1  "<pres_kPa>"
  Bus Selector4/1 -> Relational Operator/2  "<pres_kPa>"
  Bleed Valve on/off/1 -> Terminator1/1, Gain1/1, Sum2/2
  Bus Selector4/2 -> Terminator/1  "<mdot_kgps>"
  Sum2/1 -> Divide/2  "dm/dt"
  Bus Creator/1 -> Bus Selector2/1
  Gain1/1 -> Sum2/1, Bus Creator/1  "mdot_kgps"
  Gain/1 -> Bus Creator/2, Z(T,P)/2  "pres_kPa"
  Sum1/1 -> Divide/5
  resevor volume/1 -> Sum1/1
  air pres/1 -> Gain/1
  Divide/1 -> air pres/1
  Z(T,P)/1 -> Divide/4
  R_air/1 -> Divide/1
  Bus Selector4/3 -> Divide/3, Z(T,P)/1  "<temp_K>"
  Sum/1 -> mass/1  "dm/dt"
  mdot_out/1 -> Gain6/1, Sum/3  "mdot_kgps"
  Bus Selector3/2 -> Sum/1, Divide1/2  "<mdot_kgps>"
  Bypass Return/1 -> Bus Selector3/1
  mass flow off2/1 -> Divide3/2
  mass flow off3/1 -> Divide4/2
  mass flow off5/1 -> Divide4/1
  Divide4/1 -> Add/2
  Divide3/1 -> Add/1
  Add/1 -> Bleed Valve on/off1/2
  mass flow off6/1 -> Bleed Valve on/off1/3
  Bleed Valve on/off1/1 -> Sum4/2
  mass flow off4/1 -> Bleed Valve on/off1/1  "pres_kPa"
  Bus Creator2/1 -> Bus Selector4/1
  mass flow off9/1 -> Gain4/1
  mass flow off8/1 -> Gain3/1
  mass flow off7/1 -> Gain2/1
  Gain2/1 -> Bus Creator2/1  "pres_kPa"
  Gain4/1 -> Bus Creator2/3  "temp_K"
  Gain3/1 -> Bus Creator2/2  "mdot_kgps"
  Gain6/1 -> Bus Creator1/3  "mdot_kgps"
  Gain5/1 -> Bus Creator1/2  "temp_K"
  Sum4/1 -> Gain7/1  "pres_kPa"
  Gain7/1 -> Bus Creator1/1  "pres_kPa"

== system Boeing787_NewMission_ElectricalThermalHydraulicECS/Hydraulic/Right Hydraulic System/DC Speed Servo ==
  T_load (Nm) : Inport
  Speed_ref (RPM) : Inport  Port=2
  Voltage : Inport  Port=3
  DC Machine : Subsystem
  Fcn : Fcn  Expr=u(1)/(u(2)+0.1)
  Gain2 : Gain  Gain=60/(2*pi)
  Mux : Mux  Inputs=2
  PID Controller : simulink/Continuous/PID Controller  Controller=PID  TimeDomain=Continuous-time  SampleTime=-1  IntegratorMethod=Forward Euler  FilterMethod=Forward Euler  Form=Parallel  UseFilter=on  ControllerParametersSource=internal  P=1  I=0.1  D=0  N=100  InitialConditionSource=internal  InitialConditionForIntegrator=0  InitialConditionForFilter=0  ExternalReset=none  LimitOutput=off  UpperSaturationLimit=inf  LowerSaturationLimit=-inf  LinearizeAsGain=on  AntiWindupMode=none  Kb=1  TrackingMode=off  Kt=1  PParamMin=[]  PParamMax=[]  IParamMin=[]  IParamMax=[]  DParamMin=[]  DParamMax=[]  NParamMin=[]  NParamMax=[]  KbParamMin=[]  KbParamMax=[]  KtParamMin=[]  KtParamMax=[]  POutMin=[]  POutMax=[]  IOutMin=[]  IOutMax=[]  DOutMin=[]  DOutMax=[]  NOutMin=[]  NOutMax=[]  KbOutMin=[]  KbOutMax=[]  KtOutMin=[]  KtOutMax=[]  IntegratorOutMin=[]  IntegratorOutMax=[]  FilterOutMin=[]  FilterOutMax=[]  SumOutMin=[]  SumOutMax=[]  SumI1OutMin=[]  SumI1OutMax=[]  SumI2OutMin=[]  SumI2OutMax=[]  SumI3OutMin=[]  SumI3OutMax=[]  SumDOutMin=[]  SumDOutMax=[]  SaturationOutMin=[]  SaturationOutMax=[]  IntegratorContinuousStateAttributes=''  IntegratorStateMustResolveToSignalObject=off  IntegratorRTWStateStorageClass=Auto  FilterContinuousStateAttributes=''  FilterStateMustResolveToSignalObject=off  FilterRTWStateStorageClass=Auto  DifferentiatorICPrevScaledInput=0  DifferentiatorOutMin=[]  DifferentiatorOutMax=[]
  Sum : Sum  Inputs=-+|
  Terminator{,1..3} (4 alike) : Terminator
  w_m : Outport
  i_load : Outport  Port=2
  T_em : Outport  Port=3
  Ploss : Outport  Port=4
  wires:
  DC Machine/5(Plosses) -> Ploss/1
  Sum/1 -> PID Controller/1
  Gain2/1 -> Sum/1, w_m/1
  Speed_ref (RPM)/1 -> Sum/2
  T_load (Nm)/1 -> DC Machine/3(Tload)
  DC Machine/6(Te) -> T_em/1
  Mux/1 -> Fcn/1
  DC Machine/3(Pe) -> Mux/1
  Fcn/1 -> i_load/1
  DC Machine/7(Speed) -> Gain2/1
  Voltage/1 -> DC Machine/1(Vf), Mux/2
  PID Controller/1 -> DC Machine/2(Va)
  DC Machine/8(theta) -> Terminator3/1
  DC Machine/1(If) -> Terminator/1
  DC Machine/2(Ia) -> Terminator1/1
  DC Machine/4(Pm) -> Terminator2/1

== system Boeing787_NewMission_ElectricalThermalHydraulicECS/Hydraulic/Right Hydraulic System/Sinks ==
  "Motor PLoss " : Inport
  Motor Current Load : Inport  Port=2
  Out1 : Outport
  wires:
  "Motor PLoss "/1 -> Out1/1

== system Boeing787_NewMission_ElectricalThermalHydraulicECS/ECS/Left Pack/DC Speed Servo1/DC Machine ==
  note: Armature Current ia
  note: Field Current If
  Vf : Inport
  Va : Inport  Port=2
  Tload : Inport  Port=3
  Gain : Gain  Gain=Rfsh
  Gain1 : Gain  Gain=1/Lfsh
  Gain2 : Gain  Gain=Ra
  Gain3 : Gain  Gain=1/La
  Gain4 : Gain  Gain=1/J
  Gain7 : Gain  Gain=Lmsh
  Gain8 : Gain  Gain=Ra
  Gain9 : Gain  Gain=Rfsh
  Integrator : Integrator
  Integrator1 : Integrator
  Integrator2 : Integrator  InitialCondition=1  LimitOutput=on  LowerSaturationLimit=1
  Integrator3 : Integrator  ZeroCross=off
  Math Function1 : Math  Operator=square  SaturateOnIntegerOverflow=on
  Math Function2 : Math  Operator=square  SaturateOnIntegerOverflow=on
  Product{,1..4} (5 alike) : Product  RndMeth=Zero
  Scope : Scope
  Sum : Sum  Inputs=|+-
  Sum1 : Sum  Inputs=-+-
  Sum2 : Sum  Inputs=+-
  Sum4 : Sum  Inputs=|++
  Sum5 : Sum  Inputs=|++
  Terminator : Terminator
  If : Outport
  Ia : Outport  Port=2
  Pe : Outport  Port=3
  Pm : Outport  Port=4
  Plosses : Outport  Port=5
  Te : Outport  Port=6
  Speed : Outport  Port=7
  theta : Outport  Port=8
  wires:
  Integrator3/1 -> Terminator/1, theta/1
  Gain/1 -> Sum/2
  Sum/1 -> Gain1/1
  Integrator/1 -> Gain/1, [field_ct], If/1
  Sum1/1 -> Gain3/1
  Gain3/1 -> Integrator1/1
  Integrator1/1 -> Gain2/1, [arm_ct], Ia/1
  Product1/1 -> Scope/1, Sum2/1, Te/1
  Sum2/1 -> Gain4/1
  Gain4/1 -> Integrator2/1
  Gain1/1 -> Integrator/1
  Product/1 -> Sum1/1
  Gain2/1 -> Sum1/3
  [lambdaf] -> Product1/1
  [arm_ct] -> Product1/2
  [load_torque] -> Sum2/2
  [speed] -> Product/2
  [lambdaf] -> Product/1
  [field_ct] -> Gain7/1
  Gain7/1 -> [lambdaf]
  Vf/1 -> Sum/1, [vf]
  Va/1 -> Sum1/2, [va]
  [va] -> Product2/1
  [arm_ct] -> Product2/2
  Product2/1 -> Sum4/1
  [vf] -> Product3/1
  [field_ct] -> Product3/2
  Product3/1 -> Sum4/2
  Sum4/1 -> Pe/1
  [load_torque] -> Product4/1
  [speed] -> Product4/2
  Product4/1 -> Pm/1
  [arm_ct] -> Math Function1/1
  Math Function1/1 -> Gain8/1
  Gain8/1 -> Sum5/1
  [field_ct] -> Math Function2/1
  Math Function2/1 -> Gain9/1
  Gain9/1 -> Sum5/2
  Sum5/1 -> Plosses/1
  Integrator2/1 -> Speed/1, [speed], Integrator3/1
  Tload/1 -> [load_torque]

== system Boeing787_NewMission_ElectricalThermalHydraulicECS/ECS/Left Pack/DC Speed Servo2/DC Machine ==
  note: Armature Current ia
  note: Field Current If
  Vf : Inport
  Va : Inport  Port=2
  Tload : Inport  Port=3
  Gain : Gain  Gain=Rfsh
  Gain1 : Gain  Gain=1/Lfsh
  Gain2 : Gain  Gain=Ra
  Gain3 : Gain  Gain=1/La
  Gain4 : Gain  Gain=1/J
  Gain7 : Gain  Gain=Lmsh
  Gain8 : Gain  Gain=Ra
  Gain9 : Gain  Gain=Rfsh
  Integrator : Integrator
  Integrator1 : Integrator
  Integrator2 : Integrator  InitialCondition=1  LimitOutput=on  LowerSaturationLimit=1
  Integrator3 : Integrator  ZeroCross=off
  Math Function1 : Math  Operator=square  SaturateOnIntegerOverflow=on
  Math Function2 : Math  Operator=square  SaturateOnIntegerOverflow=on
  Product{,1..4} (5 alike) : Product  RndMeth=Zero
  Scope : Scope
  Sum : Sum  Inputs=|+-
  Sum1 : Sum  Inputs=-+-
  Sum2 : Sum  Inputs=+-
  Sum4 : Sum  Inputs=|++
  Sum5 : Sum  Inputs=|++
  Terminator : Terminator
  If : Outport
  Ia : Outport  Port=2
  Pe : Outport  Port=3
  Pm : Outport  Port=4
  Plosses : Outport  Port=5
  Te : Outport  Port=6
  Speed : Outport  Port=7
  theta : Outport  Port=8
  wires:
  Integrator3/1 -> Terminator/1, theta/1
  Gain/1 -> Sum/2
  Sum/1 -> Gain1/1
  Integrator/1 -> Gain/1, [field_ct], If/1
  Sum1/1 -> Gain3/1
  Gain3/1 -> Integrator1/1
  Integrator1/1 -> Gain2/1, [arm_ct], Ia/1
  Product1/1 -> Scope/1, Sum2/1, Te/1
  Sum2/1 -> Gain4/1
  Gain4/1 -> Integrator2/1
  Gain1/1 -> Integrator/1
  Product/1 -> Sum1/1
  Gain2/1 -> Sum1/3
  [lambdaf] -> Product1/1
  [arm_ct] -> Product1/2
  [load_torque] -> Sum2/2
  [speed] -> Product/2
  [lambdaf] -> Product/1
  [field_ct] -> Gain7/1
  Gain7/1 -> [lambdaf]
  Vf/1 -> Sum/1, [vf]
  Va/1 -> Sum1/2, [va]
  [va] -> Product2/1
  [arm_ct] -> Product2/2
  Product2/1 -> Sum4/1
  [vf] -> Product3/1
  [field_ct] -> Product3/2
  Product3/1 -> Sum4/2
  Sum4/1 -> Pe/1
  [load_torque] -> Product4/1
  [speed] -> Product4/2
  Product4/1 -> Pm/1
  [arm_ct] -> Math Function1/1
  Math Function1/1 -> Gain8/1
  Gain8/1 -> Sum5/1
  [field_ct] -> Math Function2/1
  Math Function2/1 -> Gain9/1
  Gain9/1 -> Sum5/2
  Sum5/1 -> Plosses/1
  Integrator2/1 -> Speed/1, [speed], Integrator3/1
  Tload/1 -> [load_torque]

== system Boeing787_NewMission_ElectricalThermalHydraulicECS/ECS/Left Pack/Primary HX (air-air)/Air_properties_in_flows_hot_and_cold ==
  In_flow_bus_hot : Inport
  In_flow_bus_cold : Inport  Port=2
  Bus Creator : BusCreator  Inputs=5
  Bus Creator3 : BusCreator  Inputs=5
  air_properties_in_cold : Subsystem
  air_properties_in_hot : Subsystem
  air_properties_in_hot1 : Outport
  air_properties_in_cold1 : Outport  Port=2
  wires:
  air_properties_in_hot/4(K_air_Wm-1K-2) -> Bus Creator/4  "K_air"
  air_properties_in_cold/5(Pr) -> Bus Creator3/5  "Pr"
  air_properties_in_hot/5(Pr) -> Bus Creator/5  "Pr"
  In_flow_bus_cold/1 -> air_properties_in_cold/1(In_flow_bus_cold)
  In_flow_bus_hot/1 -> air_properties_in_hot/1(In_flow_bus_hot)
  Bus Creator/1 -> air_properties_in_hot1/1
  Bus Creator3/1 -> air_properties_in_cold1/1
  air_properties_in_hot/3(mu_air_Pa.s) -> Bus Creator/3  "mu_air"
  air_properties_in_hot/2(cp_air_Jkg-1K-1) -> Bus Creator/2  "cp_air"
  air_properties_in_hot/1(rho_air_kgm-3) -> Bus Creator/1  "rho_air"
  air_properties_in_cold/4(K_air_Wm-1K-2) -> Bus Creator3/4  "K_air"
  air_properties_in_cold/3(mu_air_Pa.s) -> Bus Creator3/3  "mu_air"
  air_properties_in_cold/2(cp_air_Jkg-1K-1) -> Bus Creator3/2  "cp_air"
  air_properties_in_cold/1(rho_air_kgm-3) -> Bus Creator3/1  "rho_air"

== system Boeing787_NewMission_ElectricalThermalHydraulicECS/ECS/Left Pack/Primary HX (air-air)/C_T_c_av ==
  In_flow_bus : Inport
  air_properties : Inport  Port=2
  Tot_thermal_resist : Inport  Port=3
  Add : Sum
  Bus Selector : BusSelector  OutputSignals=mdot_kgps
  Bus Selector1 : BusSelector  OutputSignals=cp_air
  Constant : Constant
  Divide : Product  Inputs=***
  Divide1 : Product  Inputs=*/
  Gain : Gain  Gain=2
  C_T_c_av : Outport
  wires:
  Divide1/1 -> C_T_c_av/1
  Add/1 -> Divide1/2
  Constant/1 -> Add/2
  Gain/1 -> Divide1/1, Add/1
  Divide/1 -> Gain/1
  Bus Selector1/1 -> Divide/3  "<cp_air>"
  Bus Selector/1 -> Divide/2  "<mdot_kgps>"
  Tot_thermal_resist/1 -> Divide/1  "R_tot_c"
  In_flow_bus/1 -> Bus Selector/1
  air_properties/1 -> Bus Selector1/1

== system Boeing787_NewMission_ElectricalThermalHydraulicECS/ECS/Left Pack/Primary HX (air-air)/C_T_c_i ==
  In_flow_bus : Inport
  air_properties : Inport  Port=2
  Tot_thermal_resist : Inport  Port=3
  HX_parameters : Inport  Port=4
  Add : Sum
  Bus Selector : BusSelector  OutputSignals=mdot_kgps
  Bus Selector1 : BusSelector  OutputSignals=cp_air
  Bus Selector2 : BusSelector  OutputSignals=m_cm,cp_hx
  Constant : Constant
  Divide : Product  Inputs=***
  Divide2 : Product  Inputs=**///
  Gain : Gain  Gain=2
  Gain1 : Gain  Gain=2
  C_T_c_i : Outport
  wires:
  In_flow_bus/1 -> Bus Selector/1
  air_properties/1 -> Bus Selector1/1
  Tot_thermal_resist/1 -> Divide/1  "R_tot"
  Bus Selector/1 -> Divide/2, Divide2/1  "<mdot_kgps>"
  Bus Selector1/1 -> Divide/3, Divide2/2  "<cp_air>"
  Divide/1 -> Gain/1
  Gain/1 -> Add/1
  Constant/1 -> Add/2
  HX_parameters/1 -> Bus Selector2/1
  Bus Selector2/1 -> Divide2/3  "<m_cm>"
  Bus Selector2/2 -> Divide2/4  "<cp_hx>"
  Add/1 -> Divide2/5
  Gain1/1 -> C_T_c_i/1
  Divide2/1 -> Gain1/1

== system Boeing787_NewMission_ElectricalThermalHydraulicECS/ECS/Left Pack/Primary HX (air-air)/C_T_h_av ==
  In_flow_bus : Inport
  air_properties : Inport  Port=2
  Tot_thermal_resist : Inport  Port=3
  Add : Sum
  Bus Selector : BusSelector  OutputSignals=mdot_kgps
  Bus Selector1 : BusSelector  OutputSignals=cp_air
  Constant : Constant
  Divide : Product  Inputs=***
  Divide1 : Product  Inputs=*/
  Gain : Gain  Gain=2
  C_T_h_av : Outport
  wires:
  Divide1/1 -> C_T_h_av/1
  Add/1 -> Divide1/2
  Constant/1 -> Add/2
  Gain/1 -> Divide1/1, Add/1
  Divide/1 -> Gain/1
  Bus Selector1/1 -> Divide/3  "<cp_air>"
  Bus Selector/1 -> Divide/2  "<mdot_kgps>"
  Tot_thermal_resist/1 -> Divide/1  "R_tot_h"
  In_flow_bus/1 -> Bus Selector/1
  air_properties/1 -> Bus Selector1/1

== system Boeing787_NewMission_ElectricalThermalHydraulicECS/ECS/Left Pack/Primary HX (air-air)/C_T_h_i ==
  In_flow_bus : Inport
  air_properties : Inport  Port=2
  Tot_thermal_resist : Inport  Port=3
  HX_parameters : Inport  Port=4
  Add : Sum
  Bus Selector : BusSelector  OutputSignals=mdot_kgps
  Bus Selector1 : BusSelector  OutputSignals=cp_air
  Bus Selector2 : BusSelector  OutputSignals=m_cm,cp_hx
  Constant : Constant
  Divide : Product  Inputs=***
  Divide2 : Product  Inputs=**///
  Gain : Gain  Gain=2
  Gain1 : Gain  Gain=2
  C_T_h_i : Outport
  wires:
  Gain1/1 -> C_T_h_i/1
  Add/1 -> Divide2/5
  Bus Selector2/2 -> Divide2/4  "<cp_hx>"
  Bus Selector2/1 -> Divide2/3  "<m_cm>"
  HX_parameters/1 -> Bus Selector2/1
  Constant/1 -> Add/2
  Gain/1 -> Add/1
  Divide/1 -> Gain/1
  Bus Selector1/1 -> Divide/3, Divide2/2  "<cp_air>"
  Bus Selector/1 -> Divide/2, Divide2/1  "<mdot_kgps>"
  Tot_thermal_resist/1 -> Divide/1  "R_tot_h"
  air_properties/1 -> Bus Selector1/1
  In_flow_bus/1 -> Bus Selector/1
  Divide2/1 -> Gain1/1

== system Boeing787_NewMission_ElectricalThermalHydraulicECS/ECS/Left Pack/Primary HX (air-air)/Calculating_T_c_av ==
  T_cm : Inport
  In_flow_bus : Inport  Port=2
  C_t_c_av : Inport  Port=3
  Add1 : Sum  Inputs=-+
  Add3 : Sum
  Bus Selector : BusSelector  OutputSignals=temp_C
  Divide1 : Product  Inputs=**
  T_c_av_degreC : Outport
  wires:
  T_cm/1 -> Add3/1, Add1/1  "T_cm"
  In_flow_bus/1 -> Bus Selector/1
  Bus Selector/1 -> Add1/2  "<temp_C>"
  C_t_c_av/1 -> Divide1/2
  Add1/1 -> Divide1/1  "T_c_i - T_cm"
  Divide1/1 -> Add3/2
  Add3/1 -> T_c_av_degreC/1

== system Boeing787_NewMission_ElectricalThermalHydraulicECS/ECS/Left Pack/Primary HX (air-air)/Calculating_T_h_av ==
  T_cm : Inport
  In_flow_bus : Inport  Port=2
  C_t_h_av : Inport  Port=3
  Add1 : Sum  Inputs=-+
  Add3 : Sum
  Bus Selector : BusSelector  OutputSignals=temp_C
  Divide1 : Product  Inputs=**
  T_h_av_degreC : Outport
  wires:
  Add1/1 -> Divide1/1  "T_h_i - T_cm"
  C_t_h_av/1 -> Divide1/2
  Bus Selector/1 -> Add1/2  "<temp_C>"
  In_flow_bus/1 -> Bus Selector/1
  T_cm/1 -> Add1/1, Add3/1  "T_cm"
  Add3/1 -> T_h_av_degreC/1
  Divide1/1 -> Add3/2

== system Boeing787_NewMission_ElectricalThermalHydraulicECS/ECS/Left Pack/Primary HX (air-air)/Calculating_core_mass_temp ==
  note: dTcm/dt
  note: Tcm
  C_T_h_i : Inport
  C_T_c_i : Inport  Port=2
  C_t_cm : Inport  Port=3
  In_flow_bus_hot : Inport  Port=4
  In_flow_bus_cold : Inport  Port=5
  Add : Sum  Inputs=++-
  Bus Selector : BusSelector  OutputSignals=temp_C
  Bus Selector1 : BusSelector  OutputSignals=temp_C
  Divide : Product  Inputs=**
  Divide1 : Product  Inputs=**
  Divide2 : Product  Inputs=**
  Integrator : Integrator  InitialCondition=T_cm_0
  Core_mass_temp_C : Outport
  wires:
  Divide1/1 -> Add/3
  C_t_cm/1 -> Divide1/2
  Integrator/1 -> Core_mass_temp_C/1, Divide1/1
  Add/1 -> Integrator/1
  Divide2/1 -> Add/2
  Divide/1 -> Add/1
  Bus Selector1/1 -> Divide2/2  "<temp_C>"
  C_T_c_i/1 -> Divide2/1
  Bus Selector/1 -> Divide/2  "<temp_C>"
  C_T_h_i/1 -> Divide/1
  In_flow_bus_cold/1 -> Bus Selector1/1
  In_flow_bus_hot/1 -> Bus Selector/1

== system Boeing787_NewMission_ElectricalThermalHydraulicECS/ECS/Left Pack/Primary HX (air-air)/Colburn_J_factor_cold ==
  Fin_prameter_ratios : Inport
  Re : Inport  Port=2
  Add : Sum
  Bus Selector : BusSelector  OutputSignals=alpha_fin,delta_fin,gamma_fin
  Constant : Constant  Value=-0.5403
  Constant1 : Constant  Value=-0.1541
  Constant2 : Constant  Value=0.1499
  Constant3 : Constant  Value=-0.0678
  Constant4 : Constant  Value=1.34
  Constant5 : Constant  Value=0.504
  Constant6 : Constant  Value=0.456
  Constant7 : Constant  Value=-1.055
  Constant8 : Constant
  Constant9 : Constant  Value=0.1
  Divide : Product  Inputs=****
  Divide1 : Product  Inputs=****
  Divide2 : Product  Inputs=**
  Gain : Gain  Gain=0.6522
  Gain1 : Gain  Gain=5.269*10^(-5)
  Re1 : Math  Operator=pow  SaturateOnIntegerOverflow=on
  Re2 : Math  Operator=pow  SaturateOnIntegerOverflow=on
  alpha_fin : Math  Operator=pow  SaturateOnIntegerOverflow=on
  alpha_fin1 : Math  Operator=pow  SaturateOnIntegerOverflow=on
  delta_fin : Math  Operator=pow  SaturateOnIntegerOverflow=on
  delta_fin1 : Math  Operator=pow  SaturateOnIntegerOverflow=on
  gamma_fin : Math  Operator=pow  SaturateOnIntegerOverflow=on
  gamma_fin1 : Math  Operator=pow  SaturateOnIntegerOverflow=on
  gamma_fin2 : Math  Operator=pow  SaturateOnIntegerOverflow=on
  Colburn_J_factor : Outport
  wires:
  Divide2/1 -> Colburn_J_factor/1
  Gain/1 -> Divide2/1
  gamma_fin2/1 -> Divide2/2
  Constant9/1 -> gamma_fin2/2
  Add/1 -> gamma_fin2/1
  Gain1/1 -> Add/1
  Constant8/1 -> Add/2
  Divide1/1 -> Gain1/1
  gamma_fin1/1 -> Divide1/4
  delta_fin1/1 -> Divide1/3
  alpha_fin1/1 -> Divide1/2
  Re2/1 -> Divide1/1
  Divide/1 -> Gain/1
  gamma_fin/1 -> Divide/4
  delta_fin/1 -> Divide/3
  alpha_fin/1 -> Divide/2
  Re1/1 -> Divide/1
  Bus Selector/3 -> gamma_fin1/1, gamma_fin/1  "<gamma_fin>"
  Bus Selector/2 -> delta_fin1/1, delta_fin/1  "<delta_fin>"
  Bus Selector/1 -> alpha_fin1/1, alpha_fin/1  "<alpha_fin>"
  Re/1 -> Re2/1, Re1/1
  Constant7/1 -> gamma_fin1/2
  Constant6/1 -> delta_fin1/2
  Constant5/1 -> alpha_fin1/2
  Constant4/1 -> Re2/2
  Constant3/1 -> gamma_fin/2
  Constant2/1 -> delta_fin/2
  Constant1/1 -> alpha_fin/2
  Constant/1 -> Re1/2
  Fin_prameter_ratios/1 -> Bus Selector/1
